simulink model "model6"  (R2022a)
settings: Solver=VariableStepAuto  StartTime=0.0  StopTime=120  RelTol=1e-3
settings Model: Creator=tano-  LastModifiedBy=tano-

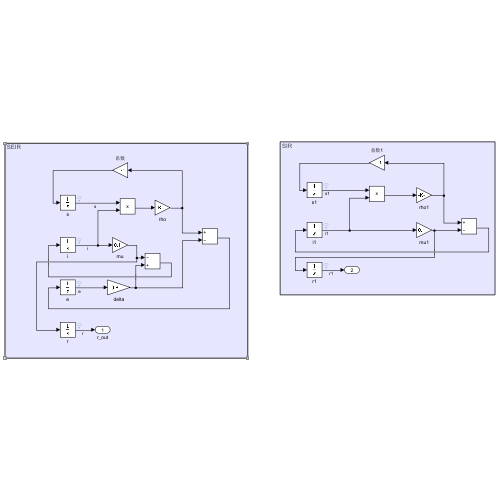
[thumbnail: Simulink's stored preview of the top-level diagram]
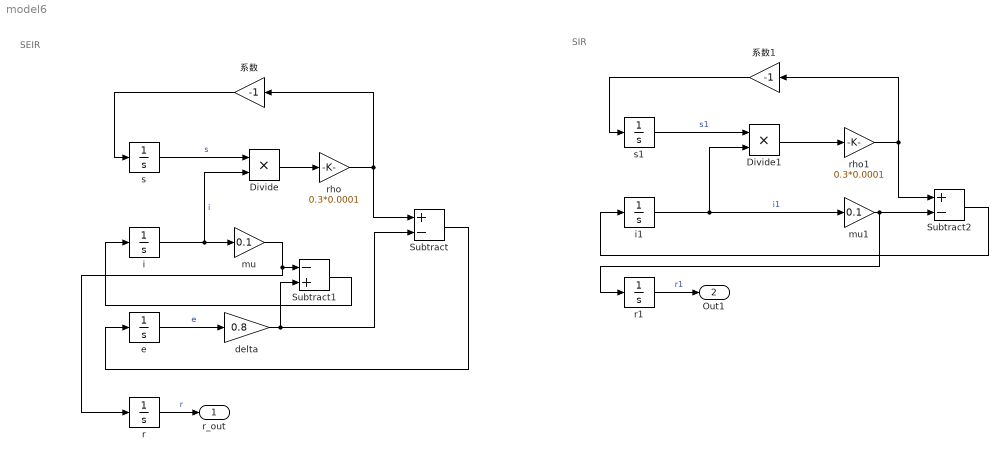
== system model6 ==
  note: SIR
  note: SEIR
  Divide : Product  Inputs=**
  Divide1 : Product  Inputs=**
  Subtract : Sum  Inputs=+-
  Subtract1 : Sum  Inputs=-+
  Subtract2 : Sum  Inputs=+-
  delta : Gain  Gain=0.8
  e : Integrator  InitialCondition=4
  i : Integrator  InitialCondition=1
  i1 : Integrator  InitialCondition=1
  mu : Gain  Gain=0.1
  mu1 : Gain  Gain=0.1
  r : Integrator
  r1 : Integrator
  rho : Gain  Gain=0.3*0.0001
  rho1 : Gain  Gain=0.3*0.0001
  s : Integrator  InitialCondition=10000
  s1 : Integrator  InitialCondition=10000
  系数 : Gain  Gain=-1
  系数1 : Gain  Gain=-1
  r_out : Outport
  Out1 : Outport  Port=2
  wires:
  i/1 -> mu/1, Divide/2  "i"
  s/1 -> Divide/1  "s"
  Divide/1 -> rho/1
  rho/1 -> Subtract/1, 系数/1
  系数/1 -> s/1
  e/1 -> delta/1  "e"
  delta/1 -> Subtract1/2, Subtract/2
  Subtract/1 -> e/1
  mu/1 -> r/1, Subtract1/1
  Subtract1/1 -> i/1
  r/1 -> r_out/1  "r"
  i1/1 -> mu1/1, Divide1/2  "i1"
  s1/1 -> Divide1/1  "s1"
  Divide1/1 -> rho1/1
  系数1/1 -> s1/1
  rho1/1 -> Subtract2/1, 系数1/1
  mu1/1 -> r1/1, Subtract2/2
  Subtract2/1 -> i1/1
  r1/1 -> Out1/1  "r1"
